simulink model "day02"  (R2026a)
settings: Solver=VariableStepAuto  StopTime=inf
libraries: simulink x1
settings Model: Creator=pete  LastModifiedBy=pete

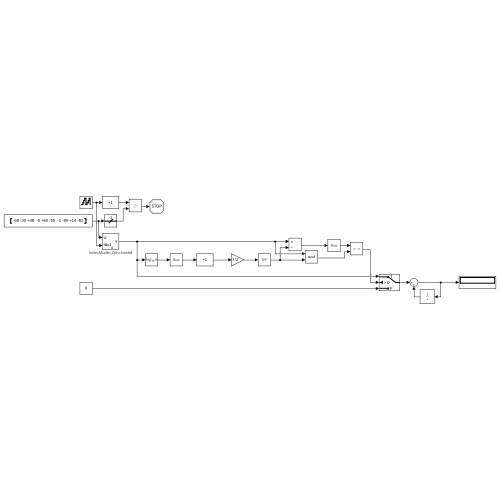
[thumbnail: Simulink's stored preview of the top-level diagram]
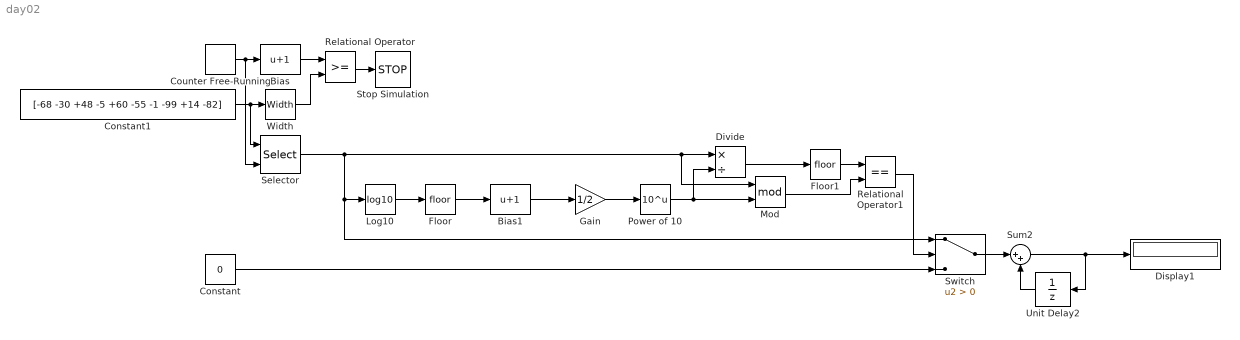
== system day02 ==
  Bias : Bias  Bias=1  SaturateOnIntegerOverflow=off
  Bias1 : Bias  Bias=1  SaturateOnIntegerOverflow=off
  Constant : Constant  Value=0
  Constant1 : Constant  Value=[-68 -30 +48 -5 +60 -55 -1 -99 +14 -82]
  Counter Free-Running : simulink/Sources/Counter Free-Running  NumBits=16  tsamp=-1
  Display1 : Display
  Divide : Product  Inputs=*/
  Floor : Rounding
  Floor1 : Rounding
  Gain : Gain  Gain=1/2
  Log10 : Math  Operator=log10
  Mod : Math  Operator=mod
  Power of 10 : Math  Operator=10^u
  Relational Operator : RelationalOperator  OutDataTypeStr=boolean  RndMeth=Simplest  InputSameDT=off
  Relational Operator1 : RelationalOperator  Operator===  OutDataTypeStr=boolean  RndMeth=Simplest  InputSameDT=off
  Selector : Selector  IndexMode=Zero-based  InputPortWidth=10  IndexOptions=Index vector (port)  Indices=[1 3]  OutputSizes=1
      settings: AttributesFormatString=IndexMode=%<IndexMode>
  Stop Simulation : Stop
  Sum2 : Sum  Inputs=|++
  Switch : Switch  Criteria=u2 > Threshold  SaturateOnIntegerOverflow=off  InputSameDT=off
  Unit Delay2 : UnitDelay  SampleTime=-1
  Width : Width
  wires:
  Counter Free-Running/1 -> Selector/2, Bias/1
  Bias/1 -> Relational Operator/1
  Relational Operator/1 -> Stop Simulation/1
  Width/1 -> Relational Operator/2
  Constant1/1 -> Selector/1, Width/1
  Log10/1 -> Floor/1
  Floor/1 -> Bias1/1
  Bias1/1 -> Gain/1
  Gain/1 -> Power of 10/1
  Selector/1 -> Switch/1, Log10/1, Divide/1, Mod/1
  Power of 10/1 -> Mod/2, Divide/2
  Divide/1 -> Floor1/1
  Floor1/1 -> Relational Operator1/1
  Mod/1 -> Relational Operator1/2
  Relational Operator1/1 -> Switch/2
  Constant/1 -> Switch/3
  Unit Delay2/1 -> Sum2/2
  Sum2/1 -> Display1/1, Unit Delay2/1
  Switch/1 -> Sum2/1
